simulink model "art_prs"  (R2020a)
settings: Solver=FixedStepAuto  StartTime=0.0  StopTime=20  FixedStep=0.01  RelTol=1e-3
undefined symbols (not defined in the file): A1, c1, c2, c3, Ca, Ce, Cv, Ed, epsilon, Es0, omega0, Ra, Re0, Rlv, Rv, Tpresion
libraries: androiduilib x6, simulink x2
settings Model: Creator=sebastian  LastModifiedBy=corte
settings OptimizationCC: EnhancedBackFolding=on  PassReuseOutputArgsAs=Individual arguments  ZeroExternalMemoryAtStartup=off  ZeroInternalMemoryAtStartup=off  MaxStackSize=64  OptimizeBlockOrder=speed  DifferentSizesBufferReuse=on  OptimizationCustomize=off  EfficientTunableParamExpr=on
settings DebuggingCC: ParameterTunabilityLossMsg=error
settings HardwareCC: ProdBitPerPointer=32  ProdBitPerSizeT=32  ProdBitPerPtrDiffT=32  ProdLargestAtomicInteger=Long  ProdLargestAtomicFloat=Double  ProdWordSize=32  ProdHWDeviceType=ARM Compatible->ARM Cortex
settings SFSimCC: MATLABDynamicMemAlloc=off
settings RTWCC: SystemTargetFile=ert.tlc  HardwareBoard=Android Device  TemplateMakefile=ert_default_tmf  RTWVerbose=off  Toolchain=Android SDK/NDK Tools
settings CodeAppCC: ForceParamTrailComments=on  IgnoreCustomStorageClasses=off  OperatorAnnotations=on  SimulinkDataObjDesc=on  SFDataObjDesc=on  InsertBlockDesc=on
settings ERTTargetCC: SupportContinuousTime=on

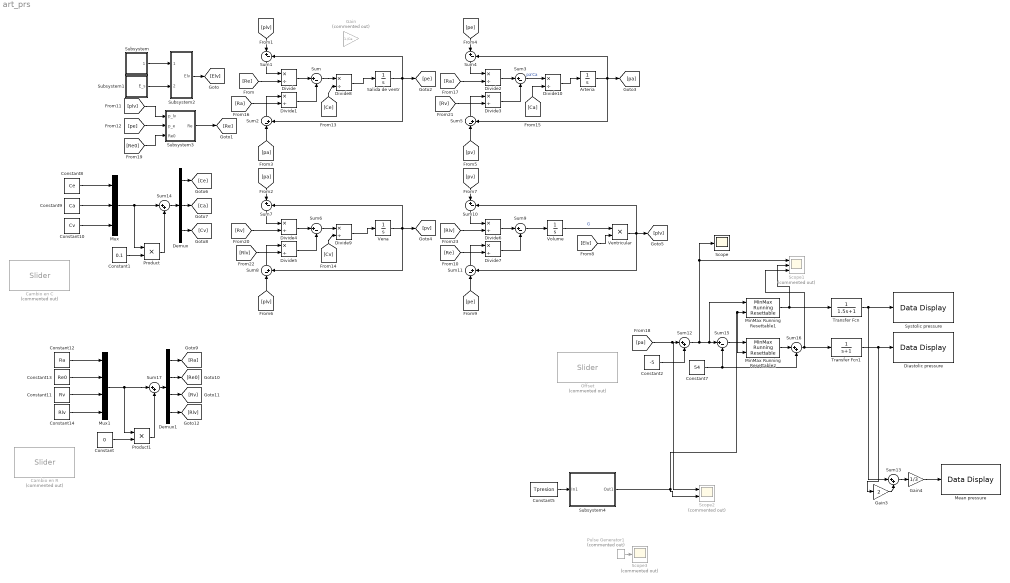
== system art_prs ==
  Arteria : Integrator  InitialCondition=55
  Cambio en C : androiduilib/Slider  Commented=on  Min=-0.3  Value=0  Max=0.4  Resolution=0.01  SliderId=art_prs/Cambio_en_C  SampleTime=0.01  BlockPlatform=Android
      settings: SourceProductBaseCode=ANDROID
  Cambio en R : androiduilib/Slider  Commented=on  Min=0  Value=0  Max=10  Resolution=0.01  SliderId=art_prs/Cambio_en_R  SampleTime=0.01  BlockPlatform=Android
      settings: SourceProductBaseCode=ANDROID
  Constant : Constant  Value=0
  Constant1 : Constant  Value=0.1
  Constant10 : Constant  Value=Cv
  Constant11 : Constant  Value=Rv
  Constant12 : Constant  Value=Ra
  Constant13 : Constant  Value=Re0
  Constant14 : Constant  Value=Rlv
  Constant2 : Constant  Value=-5
  Constant5 : Constant  Value=Tpresion
  Constant7 : Constant  Value=54
  Constant8 : Constant  Value=Ce
  Constant9 : Constant  Value=Ca
  Demux : Demux  Outputs=3
  Demux1 : Demux
  Diastolic pressure : androiduilib/Data Display  DataDisplayId=art_prs/Diastolic_pressure  Format=Integer  Precision=6  SimulateUsing=Code generation  blockPlatform=Android
      settings: SourceProductBaseCode=ANDROID
  Divide{,1..10} (11 alike) : Product  Inputs=*/
  Gain : Gain  Commented=on  Gain=1./Ce
  Gain3 : Gain  Gain=2
  Gain4 : Gain  Gain=1/3
  Mean pressure : androiduilib/Data Display  DataDisplayId=art_prs/Mean_pressure  Format=Integer  Precision=6  SimulateUsing=Code generation  blockPlatform=Android
      settings: SourceProductBaseCode=ANDROID
  MinMax Running Resettable1 : simulink/Math Operations/MinMax Running Resettable  Function=max  vinit=40
  MinMax Running Resettable2 : simulink/Math Operations/MinMax Running Resettable  Function=min  vinit=0.0
  Mux : Mux  Inputs=3
  Mux1 : Mux
  Offset : androiduilib/Slider  Commented=on  Min=-5  Value=0  Max=5  Resolution=0.01  SliderId=art_prs/Offset  SampleTime=0.01  BlockPlatform=Android
      settings: SourceProductBaseCode=ANDROID
  Product : Product
  Product1 : Product
  Pulse Generator1 : DiscretePulseGenerator  Commented=on  PulseType=Time based  Period=8  PulseWidth=0.5
  Salida de ventr : Integrator  InitialCondition=49.896
  Scope : Scope
  Scope1 : Scope  Commented=on  NumInputPorts=3
  Scope2 : Scope  Commented=on  NumInputPorts=2
  Scope3 : Scope  Commented=on
  Subsystem : Subsystem
  Subsystem1 : Subsystem
  Subsystem2 : Subsystem
  Subsystem3 : Subsystem
  Subsystem4 : Subsystem
  Sum{,1,3..4,6..7,9..10,15} (9 alike) : Sum  Inputs=|+-
  Sum{2,5,8,11} (4 alike) : Sum  Inputs=|-+
  Sum{12..14,16..17} (5 alike) : Sum  Inputs=|++
  Systolic pressure : androiduilib/Data Display  DataDisplayId=art_prs/Systolic_pressure  Format=Integer  Precision=1  SimulateUsing=Code generation  blockPlatform=Android
      settings: SourceProductBaseCode=ANDROID
  Transfer Fcn : TransferFcn  Denominator=[1.5 1]
  Transfer Fcn1 : TransferFcn  Denominator=[1 1]
  Vena : Integrator  InitialCondition=16.628
  Ventricular : Product
  Volume : Integrator  InitialCondition=49.714/0.0655
  wires:
  Subsystem/1(alpha_t) -> Subsystem2/1(alpha)
  Subsystem1/1(E_s) -> Subsystem2/2(E_s)
  Subsystem2/1(Elv) -> [Elv]
  Sum/1 -> Divide8/1
  Divide/1 -> Sum/1
  Divide1/1 -> Sum/2
  Subsystem3/1(Re) -> [Re]
  [Re] -> Divide/2
  Salida de ventr/1 -> [pe], Sum2/2, Sum1/2
  Sum1/1 -> Divide/1
  [plv] -> Sum1/1
  [Ra] -> Divide1/2
  Sum2/1 -> Divide1/1
  [pa] -> Sum2/1
  [pv] -> Sum5/1
  Sum5/1 -> Divide3/1
  [Rv] -> Divide3/2
  [pe] -> Sum4/1
  Sum4/1 -> Divide2/1
  Arteria/1 -> Sum5/2, Sum4/2, [pa]
  [Ra] -> Divide2/2
  Divide3/1 -> Sum3/2
  Divide2/1 -> Sum3/1
  Sum3/1 -> Divide10/1  "pa'Ca"
  Sum6/1 -> Divide9/1
  Divide4/1 -> Sum6/1
  Divide5/1 -> Sum6/2
  [Rv] -> Divide4/2
  Vena/1 -> [pv], Sum8/2, Sum7/2
  Sum7/1 -> Divide4/1
  [pa] -> Sum7/1
  [Rlv] -> Divide5/2
  Sum8/1 -> Divide5/1
  [plv] -> Sum8/1
  [pe] -> Sum11/1
  Sum11/1 -> Divide7/1
  [Re] -> Divide7/2
  [pv] -> Sum10/1
  Sum10/1 -> Divide6/1
  Volume/1 -> Ventricular/1  "G"
  [Rlv] -> Divide6/2
  Divide7/1 -> Sum9/2
  Divide6/1 -> Sum9/1
  Sum9/1 -> Volume/1
  Ventricular/1 -> Sum10/2, [plv], Sum11/2
  [Elv] -> Ventricular/2
  [plv] -> Subsystem3/1(p_lv)
  [pe] -> Subsystem3/2(p_e)
  Divide8/1 -> Salida de ventr/1
  Divide9/1 -> Vena/1
  Divide10/1 -> Arteria/1
  [pa] -> Scope2/1, Sum12/1
  Constant7/1 -> Sum16/2, Sum15/2
  Sum15/1 -> MinMax Running Resettable2/1
  MinMax Running Resettable2/1 -> Sum16/1
  Sum12/1 -> Scope1/1, Scope/1, MinMax Running Resettable1/1, Sum15/1
  Sum16/1 -> Scope1/3, Transfer Fcn1/1
  MinMax Running Resettable1/1 -> Scope1/2, Transfer Fcn/1
  Gain3/1 -> Sum13/2
  Sum13/1 -> Gain4/1
  Transfer Fcn1/1 -> Gain3/1, Diastolic pressure/1
  Gain4/1 -> Mean pressure/1
  Transfer Fcn/1 -> Sum13/1, Systolic pressure/1
  Constant5/1 -> Subsystem4/1(In1)
  Subsystem4/1(Out1) -> Scope2/2, MinMax Running Resettable2/2, MinMax Running Resettable1/2
  Pulse Generator1/1 -> Scope3/1
  Constant8/1 -> Mux/1
  Constant9/1 -> Mux/2
  Constant10/1 -> Mux/3
  Mux/1 -> Product/1, Sum14/1
  Product/1 -> Sum14/2
  Sum14/1 -> Demux/1
  Demux/1 -> [Ce]
  Demux/2 -> [Ca]
  Demux/3 -> [Cv]
  [Ce] -> Divide8/2
  [Cv] -> Divide9/2
  [Ca] -> Divide10/2
  Demux1/3 -> [Rv]
  Demux1/2 -> [Re0]
  Demux1/1 -> [Ra]
  Sum17/1 -> Demux1/1
  Product1/1 -> Sum17/2
  Mux1/1 -> Product1/1, Sum17/1
  Constant11/1 -> Mux1/3
  Constant13/1 -> Mux1/2
  Constant12/1 -> Mux1/1
  Constant14/1 -> Mux1/4
  Demux1/4 -> [Rlv]
  [Re0] -> Subsystem3/3(Re0)
  Constant/1 -> Product1/2
  Constant1/1 -> Product/2
  Constant2/1 -> Sum12/2

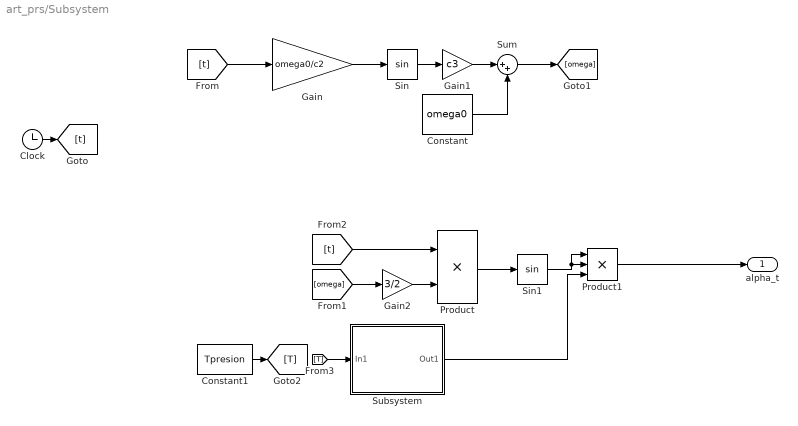
== system art_prs/Subsystem ==
  Clock : Clock
  Constant : Constant  Value=omega0
  Constant1 : Constant  Value=Tpresion
  Gain : Gain  Gain=omega0/c2
  Gain1 : Gain  Gain=c3
  Gain2 : Gain  Gain=3/2
  Product : Product
  Product1 : Product  Inputs=3
  Sin : Trigonometry
  Sin1 : Trigonometry
  Subsystem : Subsystem
  Sum : Sum  Inputs=|++
  alpha_t : Outport
  wires:
  Clock/1 -> [t]
  [t] -> Gain/1
  Gain/1 -> Sin/1
  Sin/1 -> Gain1/1
  Gain1/1 -> Sum/1
  Constant/1 -> Sum/2
  Sum/1 -> [omega]
  [t] -> Product/1
  [omega] -> Gain2/1
  Product/1 -> Sin1/1
  Sin1/1 -> Product1/1, Product1/2
  Product1/1 -> alpha_t/1
  Gain2/1 -> Product/2
  Subsystem/1(Out1) -> Product1/3
  Constant1/1 -> [T]
  [T] -> Subsystem/1(In1)

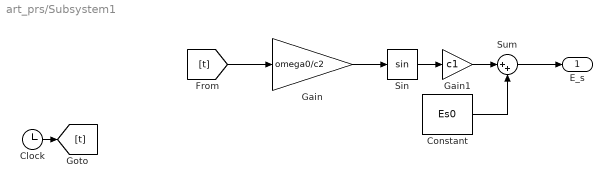
== system art_prs/Subsystem1 ==
  Clock : Clock
  Constant : Constant  Value=Es0
  Gain : Gain  Gain=omega0/c2
  Gain1 : Gain  Gain=c1
  Sin : Trigonometry
  Sum : Sum  Inputs=|++
  E_s : Outport
  wires:
  Sum/1 -> E_s/1
  Constant/1 -> Sum/2
  Gain1/1 -> Sum/1
  Sin/1 -> Gain1/1
  Gain/1 -> Sin/1
  [t] -> Gain/1
  Clock/1 -> [t]

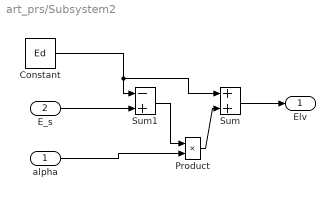
== system art_prs/Subsystem2 ==
  alpha : Inport
  E_s : Inport  Port=2
  Constant : Constant  Value=Ed
  Product : Product
  Sum : Sum
  Sum1 : Sum  Inputs=-+
  Elv : Outport
  wires:
  Constant/1 -> Sum1/1, Sum/1
  E_s/1 -> Sum1/2
  alpha/1 -> Product/2
  Sum1/1 -> Product/1
  Product/1 -> Sum/2
  Sum/1 -> Elv/1

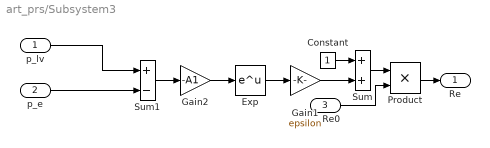
== system art_prs/Subsystem3 ==
  p_lv : Inport
  p_e : Inport  Port=2
  Re0 : Inport  Port=3
  Constant : Constant
  Exp : Math  SaturateOnIntegerOverflow=on
  Gain1 : Gain  Gain=epsilon
  Gain2 : Gain  Gain=-A1
  Product : Product
  Sum : Sum
  Sum1 : Sum  Inputs=+-
  Re : Outport
  wires:
  Sum/1 -> Product/1
  Product/1 -> Re/1
  Constant/1 -> Sum/1
  Gain1/1 -> Sum/2
  Exp/1 -> Gain1/1
  p_lv/1 -> Sum1/1
  p_e/1 -> Sum1/2
  Gain2/1 -> Exp/1
  Sum1/1 -> Gain2/1
  Re0/1 -> Product/2

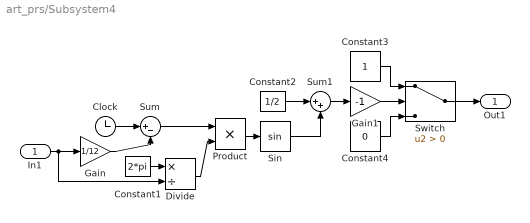
== system art_prs/Subsystem4 ==
  In1 : Inport
  Clock : Clock
  Constant1 : Constant  Value=2*pi
  Constant2 : Constant  Value=1/2
  Constant3 : Constant
  Constant4 : Constant  Value=0
  Divide : Product  Inputs=*/
  Gain : Gain  Gain=1/12
  Gain1 : Gain  Gain=-1
  Product : Product
  Sin : Trigonometry
  Sum : Sum  Inputs=|+-
  Sum1 : Sum  Inputs=|++
  Switch : Switch  Criteria=u2 > Threshold
  Out1 : Outport
  wires:
  Constant1/1 -> Divide/1
  Divide/1 -> Product/2
  Constant2/1 -> Sum1/1
  Sum/1 -> Product/1
  Gain/1 -> Sum/2
  Constant3/1 -> Switch/1
  Sum1/1 -> Gain1/1
  Sin/1 -> Sum1/2
  Constant4/1 -> Switch/3
  Gain1/1 -> Switch/2
  Product/1 -> Sin/1
  In1/1 -> Divide/2, Gain/1
  Clock/1 -> Sum/1
  Switch/1 -> Out1/1

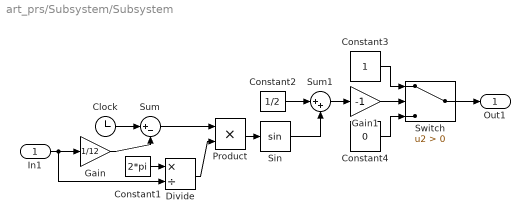
== system art_prs/Subsystem/Subsystem ==
  In1 : Inport
  Clock : Clock
  Constant1 : Constant  Value=2*pi
  Constant2 : Constant  Value=1/2
  Constant3 : Constant
  Constant4 : Constant  Value=0
  Divide : Product  Inputs=*/
  Gain : Gain  Gain=1/12
  Gain1 : Gain  Gain=-1
  Product : Product
  Sin : Trigonometry
  Sum : Sum  Inputs=|+-
  Sum1 : Sum  Inputs=|++
  Switch : Switch  Criteria=u2 > Threshold
  Out1 : Outport
  wires:
  Constant1/1 -> Divide/1
  Divide/1 -> Product/2
  Constant2/1 -> Sum1/1
  Sum/1 -> Product/1
  Gain/1 -> Sum/2
  Constant3/1 -> Switch/1
  Sum1/1 -> Gain1/1
  Sin/1 -> Sum1/2
  Constant4/1 -> Switch/3
  Gain1/1 -> Switch/2
  Product/1 -> Sin/1
  In1/1 -> Divide/2, Gain/1
  Clock/1 -> Sum/1
  Switch/1 -> Out1/1
